simulink model "Prob_3_SimuLink"  (R2012b)
settings: Solver=ode45  StartTime=0.0  StopTime=100  RelTol=1e-3
values from neighbouring files (symbols this model uses):
  A = [   0,    1,  0, 0, 0 ... (first row only)    [Prob_1.m]    (also in Prob_2.m = [            0, 1)
  B = [0;1;0;0;0]    [Prob_1.m]    (also in Prob_2.m = [0;1/((M-m)*l)])
  C = [0,0,0,1,0]    [Prob_1.m]    (also in Prob_2.m = [1,0])
  D = 0    [Prob_1.m]    (also in Prob_2.m)
  F = place(A2, B2, P)    [Prob_1.m]    (also in Prob_2.m = place(A, B, P); Prob_3.m = place(A, B, P))
  G = 1./(C2*inv(-A2+B2*F)*B2)    [Prob_1.m]    (also in Prob_2.m = 1./(C*inv(-A+B*F)*B); Prob_3.m = 1./(C*inv(-A+B*F)*B))
  L = L'    [Prob_1.m]    (also in Prob_2.m; Prob_3.m)
settings Model: Creator=Administrator  LastModifiedBy=Administrator

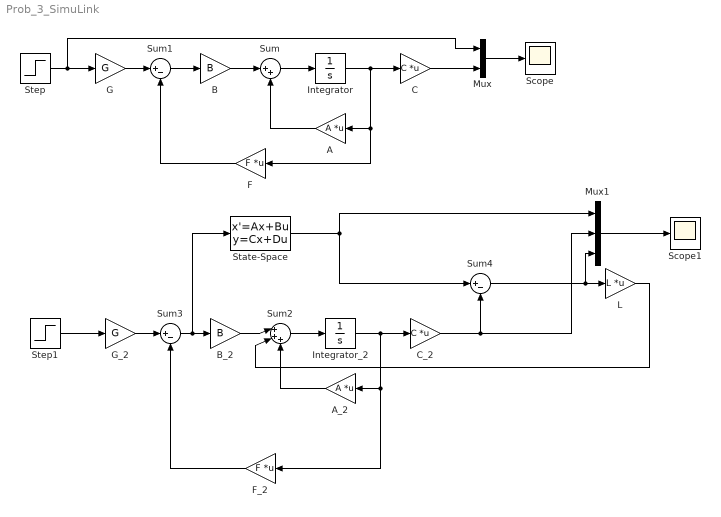
== system Prob_3_SimuLink ==
  A : Gain  Gain=A  Multiplication=Matrix(K*u)
  A_2 : Gain  Gain=A  Multiplication=Matrix(K*u)
  B : Gain  Gain=B
  B_2 : Gain  Gain=B
  C : Gain  Gain=C  Multiplication=Matrix(K*u)
  C_2 : Gain  Gain=C  Multiplication=Matrix(K*u)
  F : Gain  Gain=F  Multiplication=Matrix(K*u)
  F_2 : Gain  Gain=F  Multiplication=Matrix(K*u)
  G : Gain  Gain=G
  G_2 : Gain  Gain=G
  Integrator : Integrator
  Integrator_2 : Integrator
  L : Gain  Gain=L  Multiplication=Matrix(K*u)
  Mux : Mux  Inputs=2
  Mux1 : Mux  Inputs=3
  Scope : Scope
  Scope1 : Scope
  State-Space : StateSpace  A=A  B=B  C=C  D=D
  Step : Step  SampleTime=0
  Step1 : Step  SampleTime=0
  Sum : Sum  Inputs=|++
  Sum1 : Sum  Inputs=|+-
  Sum2 : Sum  Inputs=|+++
  Sum3 : Sum  Inputs=|+-
  Sum4 : Sum  Inputs=|+-
  wires:
  Step/1 -> Mux/1, G/1
  G/1 -> Sum1/1
  Sum1/1 -> B/1
  B/1 -> Sum/1
  Sum/1 -> Integrator/1
  Integrator/1 -> F/1, A/1, C/1
  C/1 -> Mux/2
  Mux/1 -> Scope/1
  A/1 -> Sum/2
  F/1 -> Sum1/2
  Step1/1 -> G_2/1
  G_2/1 -> Sum3/1
  Sum3/1 -> State-Space/1, B_2/1
  B_2/1 -> Sum2/1
  Sum2/1 -> Integrator_2/1
  Integrator_2/1 -> F_2/1, A_2/1, C_2/1
  A_2/1 -> Sum2/3
  F_2/1 -> Sum3/2
  L/1 -> Sum2/2
  State-Space/1 -> Sum4/1, Mux1/1
  Mux1/1 -> Scope1/1
  C_2/1 -> Mux1/2, Sum4/2
  Sum4/1 -> Mux1/3, L/1
